simulink model "unicycle"  (R2024a)
settings: Solver=ode45  StartTime=0.0  StopTime=20.0  RelTol=1e-3
undefined symbols (not defined in the file): b_reference_point, damping_coefficient, damping_coefficient_nl, k1, k2, kp1, kp2, kp3, kp4, kv, kw, natural_frequency, natural_frequency_nl, radius, x1_dest, x2_dest, x3_dest
libraries: simulink x6, robotmobilelib x3
(part 2 of 2)

== system unicycle/Unicycle Circular Trajectory Tracking via State Feedback - 1/Circular Trajectory Generation1 ==
  Mux : Mux  Inputs=3
  Trajectory generation: orientation : Subsystem
  Trajectory generation: x coordinate : Subsystem
  Trajectory generation: y coordinate : Subsystem
  desired_x : Outport
  desired_y : Outport  Port=2
  desired_theta : Outport  Port=3
  Out1 : Outport  Port=4
  wires:
  Mux/1 -> Out1/1
  Trajectory generation: x coordinate/1(xd) -> Mux/1, desired_x/1
  Trajectory generation: y coordinate/1(yd) -> Mux/2, desired_y/1
  Trajectory generation: orientation/1(Out1) -> Mux/3, desired_theta/1

== system unicycle/Unicycle Circular Trajectory Tracking via State Feedback - 1/Differential Flatness1 ==
  desired_x : Inport
  desired_y : Inport  Port=2
  desired_theta : Inport  Port=3
  Flatness : MATLAB Function  TreatAsAtomicUnit=on
  Mux : Mux  Inputs=3
  Reference trajectories derivatives : Subsystem
  Scope : Scope
  Scope1 : Scope
  qd : Outport
  vd : Outport  Port=2
  wd : Outport  Port=3
  wires:
  Flatness/1(vd_) -> Scope/1, vd/1
  Mux/1 -> qd/1
  Flatness/2(wd_) -> Scope1/1, wd/1
  desired_y/1 -> Mux/2
  desired_x/1 -> Mux/1
  desired_theta/1 -> Mux/3
  Reference trajectories derivatives/1(xdotdot) -> Flatness/1(xd_dotdot)
  Reference trajectories derivatives/2(xdot) -> Flatness/2(xd_dot)
  Reference trajectories derivatives/3(ydot) -> Flatness/3(yd_dot)
  Reference trajectories derivatives/4(ydotdot) -> Flatness/4(yd_dotdot)

== system unicycle/Unicycle Circular Trajectory Tracking via State Feedback - 1/Input Transform ==
  u1 : Inport
  u2 : Inport  Port=2
  e3 : Inport  Port=3
  vd : Inport  Port=4
  wd : Inport  Port=5
  MATLAB Function : MATLAB Function  TreatAsAtomicUnit=on
  v : Outport
  w : Outport  Port=2
  wires:
  MATLAB Function/1(v) -> v/1
  MATLAB Function/2(w) -> w/1
  u1/1 -> MATLAB Function/1(u1)
  u2/1 -> MATLAB Function/2(u2)
  vd/1 -> MATLAB Function/3(vd)
  wd/1 -> MATLAB Function/4(wd)
  e3/1 -> MATLAB Function/5(e3)

== system unicycle/Unicycle Circular Trajectory Tracking via State Feedback - 1/Linear Controller ==
  In3 : Inport
  flat1 : Inport  Port=2
  In5 : Inport  Port=3
  Input1 : Inport  Port=4
  In6 : Inport  Port=5
  Constant : Constant  Value=damping_coefficient
  Constant1 : Constant  Value=natural_frequency
  MATLAB Function1 : MATLAB Function  TreatAsAtomicUnit=on
  u3 : Outport
  u4 : Outport  Port=2
  wires:
  In5/1 -> MATLAB Function1/3(e3)
  Constant1/1 -> MATLAB Function1/7(natural_frequency)
  Input1/1 -> MATLAB Function1/5(wd)
  MATLAB Function1/2(u2) -> u4/1
  Constant/1 -> MATLAB Function1/6(damping_coefficient)
  flat1/1 -> MATLAB Function1/2(e2)
  MATLAB Function1/1(u1) -> u3/1
  In6/1 -> MATLAB Function1/4(vd)
  In3/1 -> MATLAB Function1/1(e1)

== system unicycle/Unicycle Circular Trajectory Tracking via State Feedback - 1/Non Linear Controller1 ==
  In1 : Inport
  flat : Inport  Port=2
  In4 : Inport  Port=3
  vd : Inport  Port=4
  Input : Inport  Port=5
  Constant : Constant  Value=damping_coefficient_nl
  Constant1 : Constant  Value=natural_frequency_nl
  MATLAB Function : MATLAB Function  TreatAsAtomicUnit=on
  u1 : Outport
  u2 : Outport  Port=2
  wires:
  In1/1 -> MATLAB Function/1(e1)
  MATLAB Function/1(u1) -> u1/1
  MATLAB Function/2(u2) -> u2/1
  flat/1 -> MATLAB Function/2(e2)
  In4/1 -> MATLAB Function/3(e3)
  vd/1 -> MATLAB Function/4(vd)
  Input/1 -> MATLAB Function/5(wd)
  Constant/1 -> MATLAB Function/6(damping)
  Constant1/1 -> MATLAB Function/7(natural_frequrncy)

== system unicycle/Unicycle Circular Trajectory Tracking via State Feedback - 1/Rotation matrix ==
  ew : Inport
  theta : Inport  Port=2
  MATLAB Function : MATLAB Function  TreatAsAtomicUnit=on
  Out1 : Outport
  Out2 : Outport  Port=2
  eb : Outport  Port=3
  wires:
  ew/1 -> MATLAB Function/1(ew)
  MATLAB Function/1(xb) -> Out1/1  "xb"
  MATLAB Function/2(yb) -> Out2/1  "yb"
  MATLAB Function/3(thetab) -> eb/1  "thetab"
  theta/1 -> MATLAB Function/2(theta)

== system unicycle/Unicycle Circular Trajectory Tracking via State Feedback - 2/Circular Trajectory Generation1 ==
  Mux : Mux  Inputs=3
  Trajectory generation: orientation : Subsystem
  Trajectory generation: x coordinate : Subsystem
  Trajectory generation: y coordinate : Subsystem
  desired_x : Outport
  desired_y : Outport  Port=2
  desired_theta : Outport  Port=3
  Out1 : Outport  Port=4
  wires:
  Mux/1 -> Out1/1
  Trajectory generation: x coordinate/1(xd) -> Mux/1, desired_x/1
  Trajectory generation: y coordinate/1(yd) -> Mux/2, desired_y/1
  Trajectory generation: orientation/1(Out1) -> Mux/3, desired_theta/1

== system unicycle/Unicycle Circular Trajectory Tracking via State Feedback - 2/Differential Flatness1 ==
  desired_x : Inport
  desired_y : Inport  Port=2
  desired_theta : Inport  Port=3
  Flatness : MATLAB Function  TreatAsAtomicUnit=on
  Mux : Mux  Inputs=3
  Reference trajectories derivatives : Subsystem
  Scope : Scope
  Scope1 : Scope
  qd : Outport
  vd : Outport  Port=2
  wd : Outport  Port=3
  wires:
  Flatness/1(vd_) -> Scope/1, vd/1
  Mux/1 -> qd/1
  Flatness/2(wd_) -> Scope1/1, wd/1
  desired_y/1 -> Mux/2
  desired_x/1 -> Mux/1
  desired_theta/1 -> Mux/3
  Reference trajectories derivatives/1(xdotdot) -> Flatness/1(xd_dotdot)
  Reference trajectories derivatives/2(xdot) -> Flatness/2(xd_dot)
  Reference trajectories derivatives/3(ydot) -> Flatness/3(yd_dot)
  Reference trajectories derivatives/4(ydotdot) -> Flatness/4(yd_dotdot)

== system unicycle/Unicycle Circular Trajectory Tracking via State Feedback - 2/Input Transform ==
  u1 : Inport
  u2 : Inport  Port=2
  e3 : Inport  Port=3
  vd : Inport  Port=4
  wd : Inport  Port=5
  MATLAB Function : MATLAB Function  TreatAsAtomicUnit=on
  v : Outport
  w : Outport  Port=2
  wires:
  MATLAB Function/1(v) -> v/1
  MATLAB Function/2(w) -> w/1
  u1/1 -> MATLAB Function/1(u1)
  u2/1 -> MATLAB Function/2(u2)
  vd/1 -> MATLAB Function/3(vd)
  wd/1 -> MATLAB Function/4(wd)
  e3/1 -> MATLAB Function/5(e3)

== system unicycle/Unicycle Circular Trajectory Tracking via State Feedback - 2/Linear Controller ==
  In3 : Inport
  flat1 : Inport  Port=2
  In5 : Inport  Port=3
  Input1 : Inport  Port=4
  In6 : Inport  Port=5
  Constant : Constant  Value=damping_coefficient
  Constant1 : Constant  Value=natural_frequency
  MATLAB Function1 : MATLAB Function  TreatAsAtomicUnit=on
  u3 : Outport
  u4 : Outport  Port=2
  wires:
  In5/1 -> MATLAB Function1/3(e3)
  Constant1/1 -> MATLAB Function1/7(natural_frequency)
  Input1/1 -> MATLAB Function1/5(wd)
  MATLAB Function1/2(u2) -> u4/1
  Constant/1 -> MATLAB Function1/6(damping_coefficient)
  flat1/1 -> MATLAB Function1/2(e2)
  MATLAB Function1/1(u1) -> u3/1
  In6/1 -> MATLAB Function1/4(vd)
  In3/1 -> MATLAB Function1/1(e1)

== system unicycle/Unicycle Circular Trajectory Tracking via State Feedback - 2/Non Linear Controller ==
  In1 : Inport
  flat : Inport  Port=2
  In4 : Inport  Port=3
  vd : Inport  Port=4
  Input : Inport  Port=5
  Constant : Constant  Value=damping_coefficient_nl
  Constant1 : Constant  Value=natural_frequency_nl
  MATLAB Function : MATLAB Function  TreatAsAtomicUnit=on
  u1 : Outport
  u2 : Outport  Port=2
  wires:
  In1/1 -> MATLAB Function/1(e1)
  MATLAB Function/1(u1) -> u1/1
  MATLAB Function/2(u2) -> u2/1
  flat/1 -> MATLAB Function/2(e2)
  In4/1 -> MATLAB Function/3(e3)
  vd/1 -> MATLAB Function/4(vd)
  Input/1 -> MATLAB Function/5(wd)
  Constant/1 -> MATLAB Function/6(damping)
  Constant1/1 -> MATLAB Function/7(natural_frequrncy)

== system unicycle/Unicycle Circular Trajectory Tracking via State Feedback - 2/Rotation matrix ==
  ew : Inport
  theta : Inport  Port=2
  MATLAB Function : MATLAB Function  TreatAsAtomicUnit=on
  Out1 : Outport
  Out2 : Outport  Port=2
  eb : Outport  Port=3
  wires:
  ew/1 -> MATLAB Function/1(ew)
  MATLAB Function/1(xb) -> Out1/1  "xb"
  MATLAB Function/2(yb) -> Out2/1  "yb"
  MATLAB Function/3(thetab) -> eb/1  "thetab"
  theta/1 -> MATLAB Function/2(theta)

== system unicycle/Unicycle Circular Trajectory Tracking via State Feedback - 3/Circular Trajectory Generation1 ==
  Mux : Mux  Inputs=3
  Trajectory generation: orientation : Subsystem
  Trajectory generation: x coordinate : Subsystem
  Trajectory generation: y coordinate : Subsystem
  desired_x : Outport
  desired_y : Outport  Port=2
  desired_theta : Outport  Port=3
  Out1 : Outport  Port=4
  wires:
  Mux/1 -> Out1/1
  Trajectory generation: x coordinate/1(xd) -> Mux/1, desired_x/1
  Trajectory generation: y coordinate/1(yd) -> Mux/2, desired_y/1
  Trajectory generation: orientation/1(Out1) -> Mux/3, desired_theta/1

== system unicycle/Unicycle Circular Trajectory Tracking via State Feedback - 3/Differential Flatness1 ==
  desired_x : Inport
  desired_y : Inport  Port=2
  desired_theta : Inport  Port=3
  Flatness : MATLAB Function  TreatAsAtomicUnit=on
  Mux : Mux  Inputs=3
  Reference trajectories derivatives : Subsystem
  Scope : Scope
  Scope1 : Scope
  qd : Outport
  vd : Outport  Port=2
  wd : Outport  Port=3
  wires:
  Flatness/1(vd_) -> Scope/1, vd/1
  Mux/1 -> qd/1
  Flatness/2(wd_) -> Scope1/1, wd/1
  desired_y/1 -> Mux/2
  desired_x/1 -> Mux/1
  desired_theta/1 -> Mux/3
  Reference trajectories derivatives/1(xdotdot) -> Flatness/1(xd_dotdot)
  Reference trajectories derivatives/2(xdot) -> Flatness/2(xd_dot)
  Reference trajectories derivatives/3(ydot) -> Flatness/3(yd_dot)
  Reference trajectories derivatives/4(ydotdot) -> Flatness/4(yd_dotdot)

== system unicycle/Unicycle Circular Trajectory Tracking via State Feedback - 3/Input Transform ==
  u1 : Inport
  u2 : Inport  Port=2
  e3 : Inport  Port=3
  vd : Inport  Port=4
  wd : Inport  Port=5
  MATLAB Function : MATLAB Function  TreatAsAtomicUnit=on
  v : Outport
  w : Outport  Port=2
  wires:
  MATLAB Function/1(v) -> v/1
  MATLAB Function/2(w) -> w/1
  u1/1 -> MATLAB Function/1(u1)
  u2/1 -> MATLAB Function/2(u2)
  vd/1 -> MATLAB Function/3(vd)
  wd/1 -> MATLAB Function/4(wd)
  e3/1 -> MATLAB Function/5(e3)

== system unicycle/Unicycle Circular Trajectory Tracking via State Feedback - 3/Linear Controller ==
  In3 : Inport
  flat1 : Inport  Port=2
  In5 : Inport  Port=3
  Input1 : Inport  Port=4
  In6 : Inport  Port=5
  Constant : Constant  Value=damping_coefficient
  Constant1 : Constant  Value=natural_frequency
  MATLAB Function1 : MATLAB Function  TreatAsAtomicUnit=on
  u3 : Outport
  u4 : Outport  Port=2
  wires:
  In5/1 -> MATLAB Function1/3(e3)
  Constant1/1 -> MATLAB Function1/7(natural_frequency)
  Input1/1 -> MATLAB Function1/5(wd)
  MATLAB Function1/2(u2) -> u4/1
  Constant/1 -> MATLAB Function1/6(damping_coefficient)
  flat1/1 -> MATLAB Function1/2(e2)
  MATLAB Function1/1(u1) -> u3/1
  In6/1 -> MATLAB Function1/4(vd)
  In3/1 -> MATLAB Function1/1(e1)

== system unicycle/Unicycle Circular Trajectory Tracking via State Feedback - 3/Non Linear Controller1 ==
  In1 : Inport
  flat : Inport  Port=2
  In4 : Inport  Port=3
  vd : Inport  Port=4
  Input : Inport  Port=5
  Constant : Constant  Value=damping_coefficient_nl
  Constant1 : Constant  Value=natural_frequency_nl
  MATLAB Function : MATLAB Function  TreatAsAtomicUnit=on
  u1 : Outport
  u2 : Outport  Port=2
  wires:
  In1/1 -> MATLAB Function/1(e1)
  MATLAB Function/1(u1) -> u1/1
  MATLAB Function/2(u2) -> u2/1
  flat/1 -> MATLAB Function/2(e2)
  In4/1 -> MATLAB Function/3(e3)
  vd/1 -> MATLAB Function/4(vd)
  Input/1 -> MATLAB Function/5(wd)
  Constant/1 -> MATLAB Function/6(damping)
  Constant1/1 -> MATLAB Function/7(natural_frequrncy)

== system unicycle/Unicycle Circular Trajectory Tracking via State Feedback - 3/Rotation matrix ==
  ew : Inport
  theta : Inport  Port=2
  MATLAB Function : MATLAB Function  TreatAsAtomicUnit=on
  Out1 : Outport
  Out2 : Outport  Port=2
  eb : Outport  Port=3
  wires:
  ew/1 -> MATLAB Function/1(ew)
  MATLAB Function/1(xb) -> Out1/1  "xb"
  MATLAB Function/2(yb) -> Out2/1  "yb"
  MATLAB Function/3(thetab) -> eb/1  "thetab"
  theta/1 -> MATLAB Function/2(theta)

== system unicycle/Unicycle Trajectory Tracking via Output Feedback/Subsystem ==
  In1 : Inport
  In2 : Inport  Port=2
  Demux1 : Demux  Outputs=2
  Gain : Gain  Gain=k1
  Gain1 : Gain  Gain=k2
  Mux : Mux  Inputs=2
  Sum : Sum  Inputs=++|
  pb_dot : Outport
  wires:
  Demux1/1 -> Gain/1
  Demux1/2 -> Gain1/1
  In1/1 -> Demux1/1
  Gain/1 -> Mux/1
  Gain1/1 -> Mux/2
  Mux/1 -> Sum/2
  In2/1 -> Sum/1
  Sum/1 -> pb_dot/1

== system unicycle/Unicycle Trajectory Tracking via Output Feedback/Trajectory Conversion - Point B1 ==
  x : Inport
  y : Inport  Port=2
  theta : Inport  Port=3
  Constant : Constant  Value=b_reference_point
  MATLAB Function : MATLAB Function  TreatAsAtomicUnit=on
  Mux1 : Mux  Inputs=2
  "xb, yb" : Outport
  thetab : Outport  Port=2
  wires:
  x/1 -> MATLAB Function/1(x)
  y/1 -> MATLAB Function/2(y)
  theta/1 -> MATLAB Function/3(theta)
  MATLAB Function/3(thetab) -> thetab/1
  Constant/1 -> MATLAB Function/4(b)
  MATLAB Function/2(yb) -> Mux1/2
  MATLAB Function/1(xb) -> Mux1/1
  Mux1/1 -> "xb, yb"/1

== system unicycle/Unicycle Trajectory Tracking via Output Feedback/Trajectory Conversion - To Point B ==
  d_x : Inport
  d_y : Inport  Port=2
  theta : Inport  Port=3
  Constant : Constant  Value=b_reference_point
  MATLAB Function : MATLAB Function  TreatAsAtomicUnit=on
  d_xb : Outport
  d_yb : Outport  Port=2
  wires:
  d_x/1 -> MATLAB Function/1(d_x)
  d_y/1 -> MATLAB Function/2(d_y)
  theta/1 -> MATLAB Function/3(theta)
  MATLAB Function/1(xb) -> d_xb/1
  MATLAB Function/2(yb) -> d_yb/1
  Constant/1 -> MATLAB Function/4(b)

== system unicycle/Unicycle Trajectory Tracking via Output Feedback/Trajectory Generation ==
  Mux1 : Mux  Inputs=2
  Trajectory generation: x coordinate : Subsystem
  Trajectory generation: y coordinate : Subsystem
  desired_x : Outport
  desired_y : Outport  Port=2
  Out1 : Outport  Port=3
  wires:
  Trajectory generation: y coordinate/1(yd) -> Mux1/2, desired_y/1
  Mux1/1 -> Out1/1
  Trajectory generation: x coordinate/1(xd) -> Mux1/1, desired_x/1

== system unicycle/Unicycle Trajectory Tracking via Output Feedback CHAIN form - 1/Inverse Input Transform ==
  u : Inport
  theta : Inport  Port=2
  v : Inport  Port=3
  MATLAB Function : MATLAB Function  TreatAsAtomicUnit=on
  a : Outport
  w : Outport  Port=2
  wires:
  u/1 -> MATLAB Function/1(u)
  MATLAB Function/1(a) -> a/1
  v/1 -> MATLAB Function/3(v)
  theta/1 -> MATLAB Function/2(theta)
  MATLAB Function/2(w) -> w/1

== system unicycle/Unicycle Trajectory Tracking via Output Feedback CHAIN form - 1/PD Controller ==
  e : Inport
  d_z_dot : Inport  Port=2
  Constant : Constant  Value=kp1
  Constant1 : Constant  Value=kp2
  Constant2 : Constant  Value=kp3
  Constant3 : Constant  Value=kp4
  MATLAB Function : MATLAB Function  TreatAsAtomicUnit=on
  Mux : Mux  Inputs=2
  u : Outport
  wires:
  Mux/1 -> u/1
  Constant2/1 -> MATLAB Function/5(kp3_)
  Constant/1 -> MATLAB Function/3(kp1_)
  Constant3/1 -> MATLAB Function/6(kp4_)
  Constant1/1 -> MATLAB Function/4(kp2_)
  e/1 -> MATLAB Function/1(e)
  d_z_dot/1 -> MATLAB Function/2(d_z_dot)
  MATLAB Function/1(u1) -> Mux/1
  MATLAB Function/2(u2) -> Mux/2

== system unicycle/Unicycle Trajectory Tracking via Output Feedback CHAIN form - 1/To State Z ==
  x : Inport
  y : Inport  Port=2
  Derivative1 : Derivative
  Derivative2 : Derivative
  Mux : Mux
  z : Outport
  wires:
  x/1 -> Mux/1, Derivative1/1
  y/1 -> Mux/2, Derivative2/1
  Derivative1/1 -> Mux/3
  Derivative2/1 -> Mux/4
  Mux/1 -> z/1

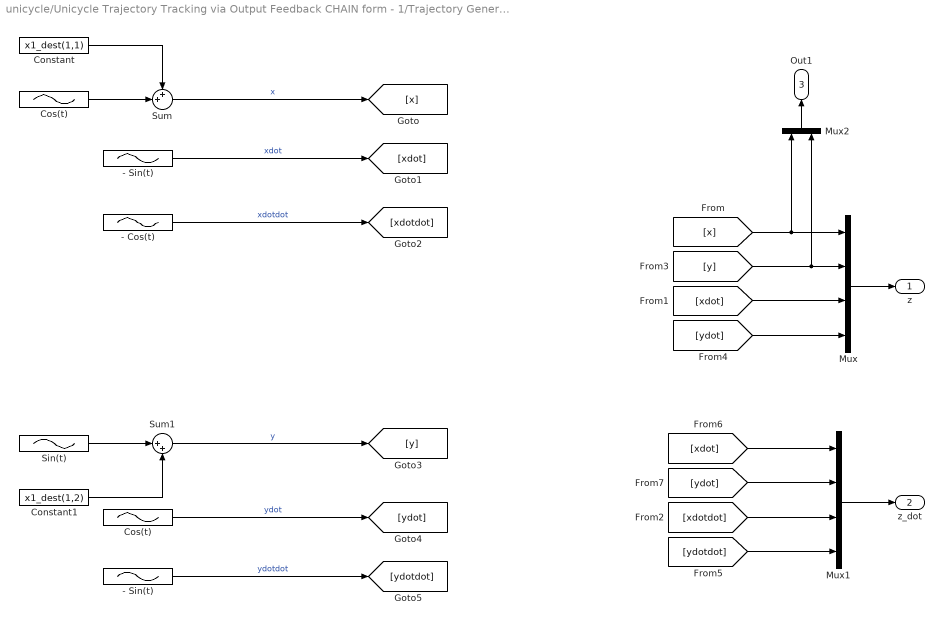
== system unicycle/Unicycle Trajectory Tracking via Output Feedback CHAIN form - 1/Trajectory Generation ==
  - Cos(t) : Sin  Amplitude=-1  Phase=pi/2  SampleTime=0
  - Sin(t) : Sin  Amplitude=-1  SampleTime=0
  "- Sin(t) " : Sin  Amplitude=-1  SampleTime=0
  Constant : Constant  Value=x1_dest(1,1)
  Constant1 : Constant  Value=x1_dest(1,2)
  Cos(t) : Sin  Phase=pi/2  SampleTime=0
  "Cos(t) " : Sin  Phase=pi/2  SampleTime=0
  Mux : Mux
  Mux1 : Mux
  Mux2 : Mux  Inputs=2
  "Sin(t) " : Sin  SampleTime=0
  Sum : Sum  Inputs=++|
  Sum1 : Sum  Inputs=|++
  z : Outport
  z_dot : Outport  Port=2
  Out1 : Outport  Port=3
  wires:
  Cos(t)/1 -> Sum/2
  Constant/1 -> Sum/1
  Sum/1 -> [x]  "x"
  "Sin(t) "/1 -> Sum1/1
  Constant1/1 -> Sum1/2
  - Sin(t)/1 -> [xdot]  "xdot"
  - Cos(t)/1 -> [xdotdot]  "xdotdot"
  Sum1/1 -> [y]  "y"
  "Cos(t) "/1 -> [ydot]  "ydot"
  "- Sin(t) "/1 -> [ydotdot]  "ydotdot"
  [x] -> Mux/1, Mux2/1
  [y] -> Mux2/2, Mux/2
  [xdot] -> Mux/3
  [ydot] -> Mux/4
  Mux/1 -> z/1
  [xdot] -> Mux1/1
  [ydot] -> Mux1/2
  [xdotdot] -> Mux1/3
  [ydotdot] -> Mux1/4
  Mux1/1 -> z_dot/1
  Mux2/1 -> Out1/1

== system unicycle/Unicycle Trajectory Tracking via Output Feedback CHAIN form - 2/Inverse Input Transform ==
  u : Inport
  theta : Inport  Port=2
  v : Inport  Port=3
  MATLAB Function : MATLAB Function  TreatAsAtomicUnit=on
  a : Outport
  w : Outport  Port=2
  wires:
  u/1 -> MATLAB Function/1(u)
  MATLAB Function/1(a) -> a/1
  v/1 -> MATLAB Function/3(v)
  theta/1 -> MATLAB Function/2(theta)
  MATLAB Function/2(w) -> w/1

== system unicycle/Unicycle Trajectory Tracking via Output Feedback CHAIN form - 2/PD Controller ==
  e : Inport
  d_z_dot : Inport  Port=2
  Constant : Constant  Value=kp1
  Constant1 : Constant  Value=kp2
  Constant2 : Constant  Value=kp3
  Constant3 : Constant  Value=kp4
  MATLAB Function : MATLAB Function  TreatAsAtomicUnit=on
  Mux : Mux  Inputs=2
  u : Outport
  wires:
  Mux/1 -> u/1
  Constant2/1 -> MATLAB Function/5(kp3_)
  Constant/1 -> MATLAB Function/3(kp1_)
  Constant3/1 -> MATLAB Function/6(kp4_)
  Constant1/1 -> MATLAB Function/4(kp2_)
  e/1 -> MATLAB Function/1(e)
  d_z_dot/1 -> MATLAB Function/2(d_z_dot)
  MATLAB Function/1(u1) -> Mux/1
  MATLAB Function/2(u2) -> Mux/2

== system unicycle/Unicycle Trajectory Tracking via Output Feedback CHAIN form - 2/To State Z ==
  x : Inport
  y : Inport  Port=2
  Derivative1 : Derivative
  Derivative2 : Derivative
  Mux : Mux
  z : Outport
  wires:
  x/1 -> Mux/1, Derivative1/1
  y/1 -> Mux/2, Derivative2/1
  Derivative1/1 -> Mux/3
  Derivative2/1 -> Mux/4
  Mux/1 -> z/1

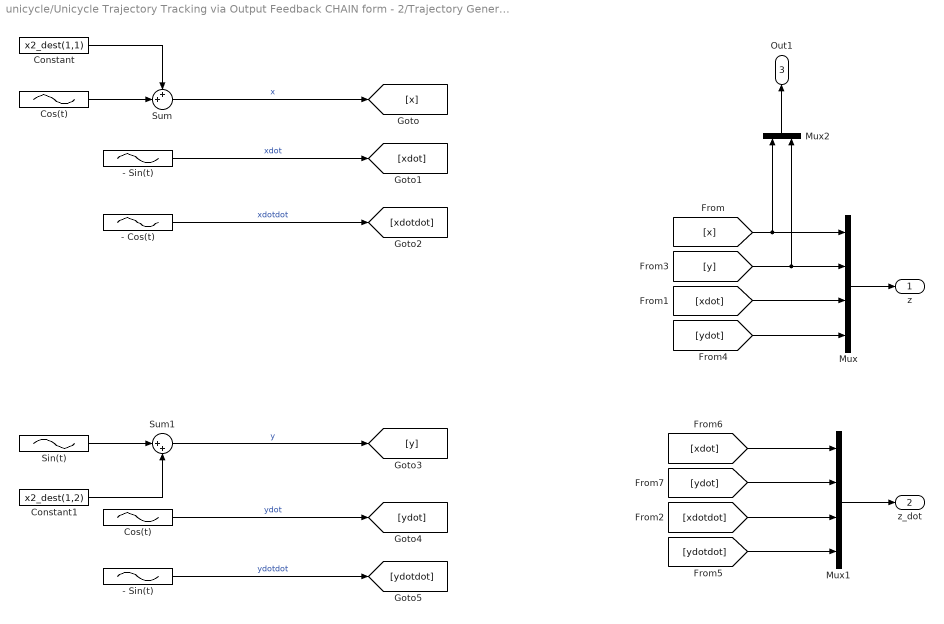
== system unicycle/Unicycle Trajectory Tracking via Output Feedback CHAIN form - 2/Trajectory Generation ==
  - Cos(t) : Sin  Amplitude=-1  Phase=pi/2  SampleTime=0
  - Sin(t) : Sin  Amplitude=-1  SampleTime=0
  "- Sin(t) " : Sin  Amplitude=-1  SampleTime=0
  Constant : Constant  Value=x2_dest(1,1)
  Constant1 : Constant  Value=x2_dest(1,2)
  Cos(t) : Sin  Phase=pi/2  SampleTime=0
  "Cos(t) " : Sin  Phase=pi/2  SampleTime=0
  Mux : Mux
  Mux1 : Mux
  Mux2 : Mux  Inputs=2
  "Sin(t) " : Sin  SampleTime=0
  Sum : Sum  Inputs=++|
  Sum1 : Sum  Inputs=|++
  z : Outport
  z_dot : Outport  Port=2
  Out1 : Outport  Port=3
  wires:
  Cos(t)/1 -> Sum/2
  Constant/1 -> Sum/1
  Sum/1 -> [x]  "x"
  "Sin(t) "/1 -> Sum1/1
  Constant1/1 -> Sum1/2
  - Sin(t)/1 -> [xdot]  "xdot"
  - Cos(t)/1 -> [xdotdot]  "xdotdot"
  Sum1/1 -> [y]  "y"
  "Cos(t) "/1 -> [ydot]  "ydot"
  "- Sin(t) "/1 -> [ydotdot]  "ydotdot"
  [x] -> Mux/1, Mux2/1
  [y] -> Mux/2, Mux2/2
  [xdot] -> Mux/3
  [ydot] -> Mux/4
  Mux/1 -> z/1
  [xdot] -> Mux1/1
  [ydot] -> Mux1/2
  [xdotdot] -> Mux1/3
  [ydotdot] -> Mux1/4
  Mux1/1 -> z_dot/1
  Mux2/1 -> Out1/1

== system unicycle/Unicycle Trajectory Tracking via Output Feedback CHAIN form - 3/Inverse Input Transform ==
  u : Inport
  theta : Inport  Port=2
  v : Inport  Port=3
  MATLAB Function : MATLAB Function  TreatAsAtomicUnit=on
  a : Outport
  w : Outport  Port=2
  wires:
  u/1 -> MATLAB Function/1(u)
  MATLAB Function/1(a) -> a/1
  v/1 -> MATLAB Function/3(v)
  theta/1 -> MATLAB Function/2(theta)
  MATLAB Function/2(w) -> w/1

== system unicycle/Unicycle Trajectory Tracking via Output Feedback CHAIN form - 3/PD Controller ==
  e : Inport
  d_z_dot : Inport  Port=2
  Constant : Constant  Value=kp1
  Constant1 : Constant  Value=kp2
  Constant2 : Constant  Value=kp3
  Constant3 : Constant  Value=kp4
  MATLAB Function : MATLAB Function  TreatAsAtomicUnit=on
  Mux : Mux  Inputs=2
  u : Outport
  wires:
  Mux/1 -> u/1
  Constant2/1 -> MATLAB Function/5(kp3_)
  Constant/1 -> MATLAB Function/3(kp1_)
  Constant3/1 -> MATLAB Function/6(kp4_)
  Constant1/1 -> MATLAB Function/4(kp2_)
  e/1 -> MATLAB Function/1(e)
  d_z_dot/1 -> MATLAB Function/2(d_z_dot)
  MATLAB Function/1(u1) -> Mux/1
  MATLAB Function/2(u2) -> Mux/2

== system unicycle/Unicycle Trajectory Tracking via Output Feedback CHAIN form - 3/To State Z ==
  x : Inport
  y : Inport  Port=2
  Derivative1 : Derivative
  Derivative2 : Derivative
  Mux : Mux
  z : Outport
  wires:
  x/1 -> Mux/1, Derivative1/1
  y/1 -> Mux/2, Derivative2/1
  Derivative1/1 -> Mux/3
  Derivative2/1 -> Mux/4
  Mux/1 -> z/1

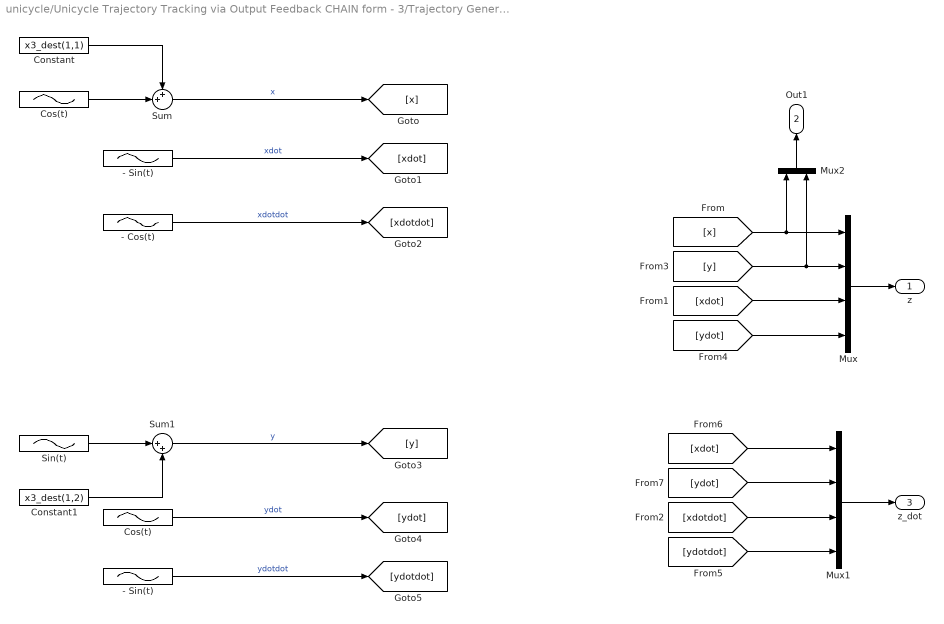
== system unicycle/Unicycle Trajectory Tracking via Output Feedback CHAIN form - 3/Trajectory Generation ==
  - Cos(t) : Sin  Amplitude=-radius  Phase=pi/2  SampleTime=0
  - Sin(t) : Sin  Amplitude=-radius  SampleTime=0
  "- Sin(t) " : Sin  Amplitude=-radius  SampleTime=0
  Constant : Constant  Value=x3_dest(1,1)
  Constant1 : Constant  Value=x3_dest(1,2)
  Cos(t) : Sin  Amplitude=radius  Phase=pi/2  SampleTime=0
  "Cos(t) " : Sin  Amplitude=radius  Phase=pi/2  SampleTime=0
  Mux : Mux
  Mux1 : Mux
  Mux2 : Mux  Inputs=2
  "Sin(t) " : Sin  Amplitude=radius  SampleTime=0
  Sum : Sum  Inputs=++|
  Sum1 : Sum  Inputs=|++
  z : Outport
  Out1 : Outport  Port=2
  z_dot : Outport  Port=3
  wires:
  Cos(t)/1 -> Sum/2
  Constant/1 -> Sum/1
  Sum/1 -> [x]  "x"
  "Sin(t) "/1 -> Sum1/1
  Constant1/1 -> Sum1/2
  - Sin(t)/1 -> [xdot]  "xdot"
  - Cos(t)/1 -> [xdotdot]  "xdotdot"
  Sum1/1 -> [y]  "y"
  "Cos(t) "/1 -> [ydot]  "ydot"
  "- Sin(t) "/1 -> [ydotdot]  "ydotdot"
  [x] -> Mux/1, Mux2/1
  [y] -> Mux2/2, Mux/2
  [xdot] -> Mux/3
  [ydot] -> Mux/4
  Mux/1 -> z/1
  [xdot] -> Mux1/1
  [ydot] -> Mux1/2
  [xdotdot] -> Mux1/3
  [ydotdot] -> Mux1/4
  Mux1/1 -> z_dot/1
  Mux2/1 -> Out1/1

== system unicycle/Unicycle Trajectory Tracking via Output Feedback1/Subsystem ==
  In1 : Inport
  In2 : Inport  Port=2
  Demux1 : Demux  Outputs=2
  Gain : Gain  Gain=k1
  Gain1 : Gain  Gain=k2
  Mux : Mux  Inputs=2
  Sum : Sum  Inputs=++|
  pb_dot : Outport
  wires:
  Demux1/1 -> Gain/1
  Demux1/2 -> Gain1/1
  In1/1 -> Demux1/1
  Gain/1 -> Mux/1
  Gain1/1 -> Mux/2
  Mux/1 -> Sum/2
  In2/1 -> Sum/1
  Sum/1 -> pb_dot/1

== system unicycle/Unicycle Trajectory Tracking via Output Feedback1/Trajectory Conversion - Point B1 ==
  x : Inport
  y : Inport  Port=2
  theta : Inport  Port=3
  Constant : Constant  Value=b_reference_point
  MATLAB Function : MATLAB Function  TreatAsAtomicUnit=on
  Mux1 : Mux  Inputs=2
  "xb, yb" : Outport
  thetab : Outport  Port=2
  wires:
  x/1 -> MATLAB Function/1(x)
  y/1 -> MATLAB Function/2(y)
  theta/1 -> MATLAB Function/3(theta)
  MATLAB Function/3(thetab) -> thetab/1
  Constant/1 -> MATLAB Function/4(b)
  MATLAB Function/2(yb) -> Mux1/2
  MATLAB Function/1(xb) -> Mux1/1
  Mux1/1 -> "xb, yb"/1

== system unicycle/Unicycle Trajectory Tracking via Output Feedback1/Trajectory Conversion - To Point B ==
  d_x : Inport
  d_y : Inport  Port=2
  theta : Inport  Port=3
  Constant : Constant  Value=b_reference_point
  MATLAB Function : MATLAB Function  TreatAsAtomicUnit=on
  d_xb : Outport
  d_yb : Outport  Port=2
  wires:
  d_x/1 -> MATLAB Function/1(d_x)
  d_y/1 -> MATLAB Function/2(d_y)
  theta/1 -> MATLAB Function/3(theta)
  MATLAB Function/1(xb) -> d_xb/1
  MATLAB Function/2(yb) -> d_yb/1
  Constant/1 -> MATLAB Function/4(b)

== system unicycle/Unicycle Trajectory Tracking via Output Feedback1/Trajectory Generation ==
  Mux1 : Mux  Inputs=2
  Trajectory generation: x coordinate : Subsystem
  Trajectory generation: y coordinate : Subsystem
  desired_x : Outport
  desired_y : Outport  Port=2
  Out1 : Outport  Port=3
  wires:
  Trajectory generation: y coordinate/1(yd) -> Mux1/2, desired_y/1
  Mux1/1 -> Out1/1
  Trajectory generation: x coordinate/1(xd) -> Mux1/1, desired_x/1

== system unicycle/Unicycle Trajectory Tracking via Output Feedback2/Subsystem ==
  In1 : Inport
  In2 : Inport  Port=2
  Demux1 : Demux  Outputs=2
  Gain : Gain  Gain=k1
  Gain1 : Gain  Gain=k2
  Mux : Mux  Inputs=2
  Sum : Sum  Inputs=++|
  pb_dot : Outport
  wires:
  Demux1/1 -> Gain/1
  Demux1/2 -> Gain1/1
  In1/1 -> Demux1/1
  Gain/1 -> Mux/1
  Gain1/1 -> Mux/2
  Mux/1 -> Sum/2
  In2/1 -> Sum/1
  Sum/1 -> pb_dot/1

== system unicycle/Unicycle Trajectory Tracking via Output Feedback2/Trajectory Conversion - Point B1 ==
  x : Inport
  y : Inport  Port=2
  theta : Inport  Port=3
  Constant : Constant  Value=b_reference_point
  MATLAB Function : MATLAB Function  TreatAsAtomicUnit=on
  Mux1 : Mux  Inputs=2
  "xb, yb" : Outport
  thetab : Outport  Port=2
  wires:
  x/1 -> MATLAB Function/1(x)
  y/1 -> MATLAB Function/2(y)
  theta/1 -> MATLAB Function/3(theta)
  MATLAB Function/3(thetab) -> thetab/1
  Constant/1 -> MATLAB Function/4(b)
  MATLAB Function/2(yb) -> Mux1/2
  MATLAB Function/1(xb) -> Mux1/1
  Mux1/1 -> "xb, yb"/1

== system unicycle/Unicycle Trajectory Tracking via Output Feedback2/Trajectory Conversion - To Point B ==
  d_x : Inport
  d_y : Inport  Port=2
  theta : Inport  Port=3
  Constant : Constant  Value=b_reference_point
  MATLAB Function : MATLAB Function  TreatAsAtomicUnit=on
  d_xb : Outport
  d_yb : Outport  Port=2
  wires:
  d_x/1 -> MATLAB Function/1(d_x)
  d_y/1 -> MATLAB Function/2(d_y)
  theta/1 -> MATLAB Function/3(theta)
  MATLAB Function/1(xb) -> d_xb/1
  MATLAB Function/2(yb) -> d_yb/1
  Constant/1 -> MATLAB Function/4(b)

== system unicycle/Unicycle Trajectory Tracking via Output Feedback2/Trajectory Generation ==
  Mux1 : Mux  Inputs=2
  Trajectory generation: x coordinate : Subsystem
  Trajectory generation: y coordinate : Subsystem
  desired_x : Outport
  desired_y : Outport  Port=2
  Out1 : Outport  Port=3
  wires:
  Trajectory generation: y coordinate/1(yd) -> Mux1/2, desired_y/1
  Mux1/1 -> Out1/1
  Trajectory generation: x coordinate/1(xd) -> Mux1/1, desired_x/1

== system unicycle/Controller Switching/Boolean Logic/If Action Subsystem ==
  In1 : Inport
  Action Port : ActionPort  ActionPortLabel=if(u1 <= rv_distance)
  Increment Stored Integer : simulink/Additional Math & Discrete/Additional Math: Increment - Decrement/Increment Stored Integer
  Out1 : Outport
  wires:
  In1/1 -> Increment Stored Integer/1
  Increment Stored Integer/1 -> Out1/1

== system unicycle/Controller Switching/Boolean Logic/If Action Subsystem1 ==
  In1 : Inport
  Action Port : ActionPort  ActionPortLabel=else
  Out1 : Outport
  wires:
  In1/1 -> Out1/1

== system unicycle/Controller Switching  /Boolean Logic/If Action Subsystem ==
  In1 : Inport
  Action Port : ActionPort  ActionPortLabel=if(u1 <= rv_distance)
  Increment Stored Integer : simulink/Additional Math & Discrete/Additional Math: Increment - Decrement/Increment Stored Integer
  Out1 : Outport
  wires:
  In1/1 -> Increment Stored Integer/1
  Increment Stored Integer/1 -> Out1/1

== system unicycle/Controller Switching  /Boolean Logic/If Action Subsystem1 ==
  In1 : Inport
  Action Port : ActionPort  ActionPortLabel=else
  Out1 : Outport
  wires:
  In1/1 -> Out1/1

== system unicycle/Controller Switching2/Boolean Logic/If Action Subsystem ==
  In1 : Inport
  Action Port : ActionPort  ActionPortLabel=if(u1 <= rv_distance)
  Increment Stored Integer : simulink/Additional Math & Discrete/Additional Math: Increment - Decrement/Increment Stored Integer
  Out1 : Outport
  wires:
  In1/1 -> Increment Stored Integer/1
  Increment Stored Integer/1 -> Out1/1

== system unicycle/Controller Switching2/Boolean Logic/If Action Subsystem1 ==
  In1 : Inport
  Action Port : ActionPort  ActionPortLabel=else
  Out1 : Outport
  wires:
  In1/1 -> Out1/1

== system unicycle/Unicycle Circular Trajectory Tracking via State Feedback - 1/Circular Trajectory Generation1/Trajectory generation: orientation ==
  Ramp : simulink/Sources/Ramp  slope=1  start=0  InitialOutput=pi/2
  Out1 : Outport
  wires:
  Ramp/1 -> Out1/1

== system unicycle/Unicycle Circular Trajectory Tracking via State Feedback - 1/Circular Trajectory Generation1/Trajectory generation: x coordinate ==
  Constant : Constant  Value=x1_dest(1,1)
  Cosinne : Sin  Amplitude=radius  Phase=pi/2  SampleTime=0
  Sum : Sum  Inputs=++|
  xd : Outport
  wires:
  Cosinne/1 -> Sum/2
  Constant/1 -> Sum/1
  Sum/1 -> xd/1  "xd"

== system unicycle/Unicycle Circular Trajectory Tracking via State Feedback - 1/Circular Trajectory Generation1/Trajectory generation: y coordinate ==
  Constant4 : Constant  Value=x1_dest(1,2)
  "Sine " : Sin  Amplitude=radius  SampleTime=0
  Sum1 : Sum  Inputs=|++
  yd : Outport
  wires:
  Sum1/1 -> yd/1  "yd"
  "Sine "/1 -> Sum1/1
  Constant4/1 -> Sum1/2

== system unicycle/Unicycle Circular Trajectory Tracking via State Feedback - 1/Differential Flatness1/Reference trajectories derivatives ==
  - Cos(t) : Sin  Amplitude=-radius  Phase=pi/2  SampleTime=0
  - Sin(t) : Sin  Amplitude=-radius  SampleTime=0
  "- Sin(t) " : Sin  Amplitude=-radius  SampleTime=0
  "Cos(t) " : Sin  Amplitude=radius  Phase=pi/2  SampleTime=0
  xdotdot : Outport
  xdot : Outport  Port=2
  ydot : Outport  Port=3
  ydotdot : Outport  Port=4
  wires:
  - Sin(t)/1 -> xdot/1  "xdot"
  - Cos(t)/1 -> xdotdot/1  "xdotdot"
  "Cos(t) "/1 -> ydot/1  "ydot"
  "- Sin(t) "/1 -> ydotdot/1  "ydotdot"

== system unicycle/Unicycle Circular Trajectory Tracking via State Feedback - 2/Circular Trajectory Generation1/Trajectory generation: orientation ==
  Ramp : simulink/Sources/Ramp  slope=1  start=0  InitialOutput=pi/2
  Out1 : Outport
  wires:
  Ramp/1 -> Out1/1

== system unicycle/Unicycle Circular Trajectory Tracking via State Feedback - 2/Circular Trajectory Generation1/Trajectory generation: x coordinate ==
  Constant : Constant  Value=x2_dest(1,1)
  Cosinne : Sin  Amplitude=radius  Phase=pi/2  SampleTime=0
  Sum : Sum  Inputs=++|
  xd : Outport
  wires:
  Cosinne/1 -> Sum/2
  Constant/1 -> Sum/1
  Sum/1 -> xd/1  "xd"

== system unicycle/Unicycle Circular Trajectory Tracking via State Feedback - 2/Circular Trajectory Generation1/Trajectory generation: y coordinate ==
  Constant4 : Constant  Value=x2_dest(1,2)
  "Sine " : Sin  Amplitude=radius  SampleTime=0
  Sum1 : Sum  Inputs=|++
  yd : Outport
  wires:
  Sum1/1 -> yd/1  "yd"
  "Sine "/1 -> Sum1/1
  Constant4/1 -> Sum1/2

== system unicycle/Unicycle Circular Trajectory Tracking via State Feedback - 2/Differential Flatness1/Reference trajectories derivatives ==
  - Cos(t) : Sin  Amplitude=-radius  Phase=pi/2  SampleTime=0
  - Sin(t) : Sin  Amplitude=-radius  SampleTime=0
  "- Sin(t) " : Sin  Amplitude=-radius  SampleTime=0
  "Cos(t) " : Sin  Amplitude=radius  Phase=pi/2  SampleTime=0
  xdotdot : Outport
  xdot : Outport  Port=2
  ydot : Outport  Port=3
  ydotdot : Outport  Port=4
  wires:
  - Sin(t)/1 -> xdot/1  "xdot"
  - Cos(t)/1 -> xdotdot/1  "xdotdot"
  "Cos(t) "/1 -> ydot/1  "ydot"
  "- Sin(t) "/1 -> ydotdot/1  "ydotdot"

== system unicycle/Unicycle Circular Trajectory Tracking via State Feedback - 3/Circular Trajectory Generation1/Trajectory generation: orientation ==
  Ramp : simulink/Sources/Ramp  slope=1  start=0  InitialOutput=pi/2
  Out1 : Outport
  wires:
  Ramp/1 -> Out1/1

== system unicycle/Unicycle Circular Trajectory Tracking via State Feedback - 3/Circular Trajectory Generation1/Trajectory generation: x coordinate ==
  Constant : Constant  Value=x3_dest(1,1)
  Cosinne : Sin  Amplitude=radius  Phase=pi/2  SampleTime=0
  Sum : Sum  Inputs=++|
  xd : Outport
  wires:
  Cosinne/1 -> Sum/2
  Constant/1 -> Sum/1
  Sum/1 -> xd/1  "xd"

== system unicycle/Unicycle Circular Trajectory Tracking via State Feedback - 3/Circular Trajectory Generation1/Trajectory generation: y coordinate ==
  Constant4 : Constant  Value=x3_dest(1,2)
  "Sine " : Sin  Amplitude=radius  SampleTime=0
  Sum1 : Sum  Inputs=|++
  yd : Outport
  wires:
  Sum1/1 -> yd/1  "yd"
  "Sine "/1 -> Sum1/1
  Constant4/1 -> Sum1/2

== system unicycle/Unicycle Circular Trajectory Tracking via State Feedback - 3/Differential Flatness1/Reference trajectories derivatives ==
  - Cos(t) : Sin  Amplitude=-radius  Phase=pi/2  SampleTime=0
  - Sin(t) : Sin  Amplitude=-radius  SampleTime=0
  "- Sin(t) " : Sin  Amplitude=-radius  SampleTime=0
  "Cos(t) " : Sin  Amplitude=radius  Phase=pi/2  SampleTime=0
  xdotdot : Outport
  xdot : Outport  Port=2
  ydot : Outport  Port=3
  ydotdot : Outport  Port=4
  wires:
  - Sin(t)/1 -> xdot/1  "xdot"
  - Cos(t)/1 -> xdotdot/1  "xdotdot"
  "Cos(t) "/1 -> ydot/1  "ydot"
  "- Sin(t) "/1 -> ydotdot/1  "ydotdot"

== system unicycle/Unicycle Trajectory Tracking via Output Feedback/Trajectory Generation/Trajectory generation: x coordinate ==
  Constant : Constant  Value=x1_dest(1,1)
  Cosinne : Sin  Amplitude=radius  Phase=pi/2  SampleTime=0
  Sum : Sum  Inputs=++|
  xd : Outport
  wires:
  Cosinne/1 -> Sum/2
  Constant/1 -> Sum/1
  Sum/1 -> xd/1  "xd"

== system unicycle/Unicycle Trajectory Tracking via Output Feedback/Trajectory Generation/Trajectory generation: y coordinate ==
  Constant1 : Constant  Value=x1_dest(1,2)
  "Sine " : Sin  Amplitude=radius  SampleTime=0
  Sum1 : Sum  Inputs=|++
  yd : Outport
  wires:
  Sum1/1 -> yd/1  "yd"
  "Sine "/1 -> Sum1/1
  Constant1/1 -> Sum1/2

== system unicycle/Unicycle Trajectory Tracking via Output Feedback1/Trajectory Generation/Trajectory generation: x coordinate ==
  Constant : Constant  Value=x3_dest(1,1)
  Cosinne : Sin  Amplitude=radius  Phase=pi/2  SampleTime=0
  Sum : Sum  Inputs=++|
  xd : Outport
  wires:
  Cosinne/1 -> Sum/2
  Constant/1 -> Sum/1
  Sum/1 -> xd/1  "xd"

== system unicycle/Unicycle Trajectory Tracking via Output Feedback1/Trajectory Generation/Trajectory generation: y coordinate ==
  Constant1 : Constant  Value=x3_dest(1,2)
  "Sine " : Sin  Amplitude=radius  SampleTime=0
  Sum1 : Sum  Inputs=|++
  yd : Outport
  wires:
  Sum1/1 -> yd/1  "yd"
  "Sine "/1 -> Sum1/1
  Constant1/1 -> Sum1/2

== system unicycle/Unicycle Trajectory Tracking via Output Feedback2/Trajectory Generation/Trajectory generation: x coordinate ==
  Constant : Constant  Value=x2_dest(1,1)
  Cosinne : Sin  Amplitude=radius  Phase=pi/2  SampleTime=0
  Sum : Sum  Inputs=++|
  xd : Outport
  wires:
  Cosinne/1 -> Sum/2
  Constant/1 -> Sum/1
  Sum/1 -> xd/1  "xd"

== system unicycle/Unicycle Trajectory Tracking via Output Feedback2/Trajectory Generation/Trajectory generation: y coordinate ==
  Constant1 : Constant  Value=x2_dest(1,2)
  "Sine " : Sin  Amplitude=radius  SampleTime=0
  Sum1 : Sum  Inputs=|++
  yd : Outport
  wires:
  Sum1/1 -> yd/1  "yd"
  "Sine "/1 -> Sum1/1
  Constant1/1 -> Sum1/2

== matlab function unicycle/Unicycle Cartesian Regulation - 2/Regulation Controller1 ==
  data: theta input; v output; w output; e input; kv input; kw input
function [v,w] = fcn(theta, e, kv, kw)

%k= sign(-(e(1)));

% linear velocity controller
v= kv*(e(1)*cos(theta) + e(2)*sin(theta));
w= kw*( atan2(-e(2), -e(1)) +(pi) - theta);

== matlab function unicycle/Unicycle Circular Trajectory Tracking via State Feedback - 2/Input Transform/MATLAB Function ==
  data: u1 input; v output; u2 input; vd input; wd input; w output; e3 input
function [v, w] = fcn(u1, u2, vd, wd, e3)

v= vd*cos(e3)- u1;
w= wd-u2;

== matlab function unicycle/Unicycle Trajectory Tracking via Output Feedback1/MATLAB Function ==
  data: v output; pb_dot input; b input; w output; theta input
function [v, w] = fcn(pb_dot, b, theta)

xb_dot= pb_dot(1);
yb_dot= pb_dot(2);

v= xb_dot*cos(theta) + yb_dot*sin(theta);

w= xb_dot*(-sin(theta)/b) + yb_dot*(cos(theta)/b);

== matlab function unicycle/Unicycle Circular Trajectory Tracking via State Feedback - 2/Linear Controller/MATLAB Function1 ==
  data: e1 input; u1 output; u2 output; e2 input; e3 input; vd input; wd input; damping_coefficient input; natural_frequency input
function [u1,  u2] = fcn(e1, e2, e3, vd, wd, damping_coefficient, natural_frequency)

csi= damping_coefficient;
a= natural_frequency;

k1= 2*csi*a;
k2= (a^2 - wd^2)/vd;
k3= k1;

u1= -k1*e1;
u2= -k2*e2 - k3*e3;

== matlab function unicycle/Unicycle Circular Trajectory Tracking via State Feedback - 2/Non Linear Controller/MATLAB Function ==
  data: e1 input; u1 output; u2 output; e2 input; e3 input; vd input; wd input; damping input; natural_frequrncy input
function [u1,  u2] = fcn(e1, e2, e3, vd, wd, damping, natural_frequrncy)

csi= damping; 
a= natural_frequrncy;

k1= 2*csi*sqrt(a*vd - wd^2);
k3= k1;
k2=a;

u1= -k1*e1;
u2= -k2*(vd* (sin(e3)/e3) )*e2 - (k3*e3);

== matlab function unicycle/Unicycle Cartesian Regulation - 3/Regulation Controller1 ==
  data: theta input; v output; w output; e input; kv input; kw input
function [v,w] = fcn(theta, e, kv, kw)

% linear velocity controller
v= kv*(e(1)*cos(theta) + e(2)*sin(theta));
w= kw*( atan2(-e(2), -e(1)) +(1*pi) - theta);

== matlab function unicycle/Unicycle Circular Trajectory Tracking via State Feedback - 1/Linear Controller/MATLAB Function1 ==
  data: e1 input; u1 output; u2 output; e2 input; e3 input; vd input; wd input; damping_coefficient input; natural_frequency input
function [u1,  u2] = fcn(e1, e2, e3, vd, wd, damping_coefficient, natural_frequency)

    csi= damping_coefficient;
    a= natural_frequency;
    
    k1= 2*csi*a;
    k2= ((a^2) - (wd^2))/vd;
    k3= k1;
    
    u1= -k1*e1;
    u2= -k2*e2 - k3*e3;
end

== matlab function unicycle/Unicycle Trajectory Tracking via Output Feedback1/Trajectory Conversion - Point B1/MATLAB Function ==
  data: x input; xb output; y input; theta input; yb output; thetab output; b input
function [xb, yb, thetab] = fcn(x, y, theta, b)

xb= x + b*cos(theta);
yb= y + b*sin(theta);
thetab= theta;

== matlab function unicycle/Unicycle Circular Trajectory Tracking via State Feedback - 2/Rotation matrix/MATLAB Function ==
  data: ew input; xb output; theta input; yb output; thetab output
function [xb, yb, thetab] = fcn(ew, theta)


xb=  cos(theta)*ew(1) + sin(theta)*ew(2);
yb= -sin(theta)*ew(1) + cos(theta)*ew(2);
thetab= ew(3);

== matlab function unicycle/Unicycle Trajectory Tracking via Output Feedback1/Trajectory Conversion - To Point B/MATLAB Function ==
  data: d_x input; xb output; d_y input; theta input; yb output; b input
function [xb, yb] = fcn(d_x, d_y, theta, b)

xb= d_x + b*cos(theta);
yb= d_y + b*sin(theta);

== matlab function unicycle/Unicycle Trajectory Tracking via Output Feedback2/MATLAB Function ==
  data: v output; pb_dot input; b input; w output; theta input
function [v, w] = fcn(pb_dot, b, theta)
    
    xb_dot= pb_dot(1);
    yb_dot= pb_dot(2);
    
    v= xb_dot*cos(theta) + yb_dot*sin(theta);
    
    w= xb_dot*(-sin(theta)/b) + yb_dot*(cos(theta)/b);
end

== matlab function unicycle/Unicycle Trajectory Tracking via Output Feedback2/Trajectory Conversion - Point B1/MATLAB Function ==
  data: x input; xb output; y input; theta input; yb output; thetab output; b input
function [xb, yb, thetab] = fcn(x, y, theta, b)

xb= x + b*cos(theta);
yb= y + b*sin(theta);
thetab= theta;

== matlab function unicycle/Unicycle Trajectory Tracking via Output Feedback2/Trajectory Conversion - To Point B/MATLAB Function ==
  data: d_x input; xb output; d_y input; theta input; yb output; b input
function [xb, yb] = fcn(d_x, d_y, theta, b)

xb= d_x + b*cos(theta);
yb= d_y + b*sin(theta);

== matlab function unicycle/Unicycle Trajectory Tracking via Output Feedback CHAIN form - 2/PD Controller/MATLAB Function ==
  data: e input; u1 output; d_z_dot input; u2 output; kp1_ input; kp2_ input; kp3_ input; kp4_ input
function [u1, u2] = fcn(e, d_z_dot, kp1_, kp2_, kp3_, kp4_)

kp1= kp1_;
kp2= kp2_;

kp3= kp3_;
kp4= kp4_;

u1= kp1*(e(1)) + kp3*(e(3)) + d_z_dot(3);
u2= kp2*(e(2)) + kp4*(e(4)) + d_z_dot(4);

== matlab function unicycle/Unicycle Trajectory Tracking via Output Feedback CHAIN form - 3/PD Controller/MATLAB Function ==
  data: e input; u1 output; d_z_dot input; u2 output; kp1_ input; kp2_ input; kp3_ input; kp4_ input
function [u1, u2] = fcn(e, d_z_dot, kp1_, kp2_, kp3_, kp4_)

kp1= kp1_;
kp2= kp2_;

kp3= kp3_;
kp4= kp4_;

u1= kp1*e(1) + kp3*e(3) + d_z_dot(3);
u2= kp2*e(2) + kp4*e(4) + d_z_dot(4);

== matlab function unicycle/Unicycle Trajectory Tracking via Output Feedback/MATLAB Function ==
  data: v output; pb_dot input; b input; w output; theta input
function [v, w] = fcn(pb_dot, b, theta)

xb_dot= pb_dot(1);
yb_dot= pb_dot(2);

v= xb_dot*cos(theta) + yb_dot*sin(theta);

w= xb_dot*(-sin(theta)/b) + yb_dot*(cos(theta)/b);

== matlab function unicycle/Unicycle Trajectory Tracking via Output Feedback/Trajectory Conversion - Point B1/MATLAB Function ==
  data: x input; xb output; y input; theta input; yb output; thetab output; b input
function [xb, yb, thetab] = fcn(x, y, theta, b)

xb= x + b*cos(theta);
yb= y + b*sin(theta);
thetab= theta;

== matlab function unicycle/Unicycle Trajectory Tracking via Output Feedback/Trajectory Conversion - To Point B/MATLAB Function ==
  data: d_x input; xb output; d_y input; theta input; yb output; b input
function [xb, yb] = fcn(d_x, d_y, theta, b)

xb= d_x + b*cos(theta);
yb= d_y + b*sin(theta);

== matlab function unicycle/Unicycle Trajectory Tracking via Output Feedback CHAIN form - 1/Inverse Input Transform/MATLAB Function ==
  data: a output; u input; theta input; v input; w output
function [a, w] = fcn(u, theta, v)

u1= u(1);
u2= u(2);

a= u1*cos(theta) + u2*sin(theta);

% if the uncycle is already inside the small circle then it start with 
% tracking and hence v=0. This implies omega to be infinite, so in this
% case let appproximate the output w
if v<=0.05
    w= u1*(-sin(theta)/0.1) + u2*(cos(theta)/0.1);
else
    w= u1*(-sin(theta)/v) + u2*(cos(theta)/v);
end

== matlab function unicycle/Unicycle Trajectory Tracking via Output Feedback CHAIN form - 3/Inverse Input Transform/MATLAB Function ==
  data: a output; u input; theta input; v input; w output
function [a, w] = fcn(u, theta, v)

u1= u(1);
u2= u(2);

a= u1*cos(theta) + u2*sin(theta);

% if the uncycle is already inside the small circle then it start with 
% tracking and hence v=0. This implies omega to be infinite, so in this
% case let appproximate the output w
if v<=0.01
    w= u1*-theta + u2;
else
    w= -u1*(sin(theta)/v) + u2*(cos(theta)/v);
end

== matlab function unicycle/Controller Switching  /Boolean Logic/Compute the distance  ==
  data: e input; e_l output
function e_l  = fcn(e)
e_l= sqrt(e(1)^2+ e(2)^2);

== matlab function unicycle/Unicycle Circular Trajectory Tracking via State Feedback - 1/Differential Flatness1/Flatness ==
  data: xd_dotdot input; xd_dot input; yd_dot input; vd_ output; wd_ output; yd_dotdot input
function [vd_, wd_] = fcn(xd_dotdot, xd_dot, yd_dot, yd_dotdot)


vd_= sqrt((xd_dot^2) + (yd_dot^2));

wd_num= (xd_dot*yd_dotdot) - (xd_dotdot*yd_dot);

wd_den= xd_dot^2 + yd_dot^2;

wd_= wd_num/wd_den;

== matlab function unicycle/Unicycle Circular Trajectory Tracking via State Feedback - 3/Differential Flatness1/Flatness ==
  data: xd_dotdot input; xd_dot input; yd_dot input; vd_ output; wd_ output; yd_dotdot input
function [vd_, wd_] = fcn(xd_dotdot, xd_dot, yd_dot, yd_dotdot)


vd_= sqrt((xd_dot^2) + (yd_dot^2));

wd_num= (xd_dot*yd_dotdot) - (xd_dotdot*yd_dot);

wd_den= xd_dot^2 + yd_dot^2;

wd_= wd_num/wd_den;

== matlab function unicycle/Unicycle Circular Trajectory Tracking via State Feedback - 3/Input Transform/MATLAB Function ==
  data: u1 input; v output; u2 input; vd input; wd input; w output; e3 input
function [v, w] = fcn(u1, u2, vd, wd, e3)

v= vd*cos(e3)- u1;
w= wd-u2;

== matlab function unicycle/Unicycle Circular Trajectory Tracking via State Feedback - 3/Linear Controller/MATLAB Function1 ==
  data: e1 input; u1 output; u2 output; e2 input; e3 input; vd input; wd input; damping_coefficient input; natural_frequency input
function [u1,  u2] = fcn(e1, e2, e3, vd, wd, damping_coefficient, natural_frequency)

csi= damping_coefficient;
a= natural_frequency;

k1= 2*csi*a;
k2= (a^2 - wd^2)/vd;
k3= k1;

u1= -k1*e1;
u2= -k2*e2 - k3*e3;

== matlab function unicycle/Unicycle Trajectory Tracking via Output Feedback CHAIN form - 1/PD Controller/MATLAB Function ==
  data: e input; u1 output; d_z_dot input; u2 output; kp1_ input; kp2_ input; kp3_ input; kp4_ input
function [u1, u2] = fcn(e, d_z_dot, kp1_, kp2_, kp3_, kp4_)

kp1= kp1_;
kp2= kp2_;

kp3= kp3_;
kp4= kp4_;

u1= kp1*(e(1)) + kp3*(e(3)) + d_z_dot(3);
u2= kp2*(e(2)) + kp4*(e(4)) + d_z_dot(4);

== matlab function unicycle/Unicycle Trajectory Tracking via Output Feedback CHAIN form - 2/Inverse Input Transform/MATLAB Function ==
  data: a output; u input; theta input; v input; w output
function [a, w] = fcn(u, theta, v)

u1= u(1);
u2= u(2);

a= u1*cos(theta) + u2*sin(theta);

% if the uncycle is already inside the small circle then it start with 
% tracking and hence v=0. This implies omega to be infinite, so in this
% case let appproximate the output w
if v<=0.05
    w= u1*-theta + u2;
else
    w= u1*(-sin(theta)/v) + u2*(cos(theta)/v);
end

== matlab function unicycle/Unicycle Cartesian Regulation - 1/Regulation Controller1 ==
  data: theta input; v output; w output; e input; kv input; kw input
function [v,w] = fcn(theta, e, kv, kw)

%k= sign(-(e(1)));

% linear velocity controller
v= kv*(e(1)*cos(theta) + e(2)*sin(theta));
w= kw*( atan2(-e(2), -e(1)) +(pi) - theta);

== matlab function unicycle/Unicycle Circular Trajectory Tracking via State Feedback - 3/Non Linear Controller1/MATLAB Function ==
  data: e1 input; u1 output; u2 output; e2 input; e3 input; vd input; wd input; damping input; natural_frequrncy input
function [u1,  u2] = fcn(e1, e2, e3, vd, wd, damping, natural_frequrncy)

csi= damping; 
a= natural_frequrncy;

k1= 2*csi*sqrt(a*vd - wd^2);
k3= k1;
k2=a;

u1= -k1*e1;
u2= -k2*(vd* (sin(e3)/e3) )*e2 - (k3*e3);

== matlab function unicycle/Unicycle Circular Trajectory Tracking via State Feedback - 3/Rotation matrix/MATLAB Function ==
  data: ew input; xb output; theta input; yb output; thetab output
function [xb, yb, thetab] = fcn(ew, theta)


xb=  cos(theta)*ew(1) + sin(theta)*ew(2);
yb= -sin(theta)*ew(1) + cos(theta)*ew(2);
thetab= ew(3);

== matlab function unicycle/Controller Switching2/Boolean Logic/Compute the distance  ==
  data: e input; e_l output
function e_l  = fcn(e)
e_l= sqrt(e(1)^2+ e(2)^2);

== matlab function unicycle/Controller Switching/Boolean Logic/Compute the distance  ==
  data: e input; e_l output
function e_l  = fcn(e)
e_l= sqrt(e(1)^2+ e(2)^2);

== matlab function unicycle/Unicycle Circular Trajectory Tracking via State Feedback - 1/Non Linear Controller1/MATLAB Function ==
  data: e1 input; u1 output; u2 output; e2 input; e3 input; vd input; wd input; damping input; natural_frequrncy input
function [u1,  u2] = fcn(e1, e2, e3, vd, wd, damping, natural_frequrncy)

csi= damping; 
a= natural_frequrncy;

k1= 2*csi*sqrt(a*vd - wd^2);
k3= k1;
k2=a;

u1= -k1*e1;
u2= -k2*(vd* (sin(e3)/e3) )*e2 - (k3*e3);

== matlab function unicycle/Unicycle Circular Trajectory Tracking via State Feedback - 1/Rotation matrix/MATLAB Function ==
  data: ew input; xb output; theta input; yb output; thetab output
function [xb, yb, thetab] = fcn(ew, theta)


xb=  cos(theta)*ew(1) + sin(theta)*ew(2);
yb= -sin(theta)*ew(1) + cos(theta)*ew(2);
thetab= ew(3);

== matlab function unicycle/Unicycle Circular Trajectory Tracking via State Feedback - 2/Differential Flatness1/Flatness ==
  data: xd_dotdot input; xd_dot input; yd_dot input; vd_ output; wd_ output; yd_dotdot input
function [vd_, wd_] = fcn(xd_dotdot, xd_dot, yd_dot, yd_dotdot)


vd_= sqrt((xd_dot^2) + (yd_dot^2));

wd_num= (xd_dot*yd_dotdot) - (xd_dotdot*yd_dot);

wd_den= xd_dot^2 + yd_dot^2;

wd_= wd_num/wd_den;

== matlab function unicycle/Unicycle Circular Trajectory Tracking via State Feedback - 1/Input Transform/MATLAB Function ==
  data: u1 input; v output; u2 input; vd input; wd input; w output; e3 input
function [v, w] = fcn(u1, u2, vd, wd, e3)

v= vd*cos(e3)- u1;
w= wd-u2;
